simulink model "UAV3D_visualizeBoxObstacle"  (Simulink 8.6)
settings: Solver=ode1  StartTime=0.0  StopTime=inf  FixedStep=1/100  RelTol=1e-6
libraries: uavsimBlockset_UAV3D_visualizeBox x2
settings Model: Creator=j.bolting  LastModifiedBy=j.bolting
settings SolverCC: AutoInsertRateTranBlk=on
settings DataIOCC: SaveFormat=Dataset  SignalLoggingSaveFormat=Dataset
settings OptimizationCC: ExpressionDepthLimit=128
settings DebuggingCC: UnderspecifiedInitializationDetection=Simplified  MergeDetectMultiDrivingBlocksExec=error  SolverPrmCheckMsg=none  FcnCallInpInsideContextMsg=EnableAllAsError  StateNameClashWarn=none
settings HardwareCC: ProdBitPerPointer=64  ProdLargestAtomicFloat=Float  ProdIntDivRoundTo=Zero  ProdEndianess=LittleEndian  ProdWordSize=64  ProdHWDeviceType=Intel->x86-64 (Windows64)
settings GRTTargetCC: GeneratePreprocessorConditionals=Use local settings  CombineOutputUpdateFcns=on  GRTInterface=off
settings ConfigComp: CovModelRefEnable=off

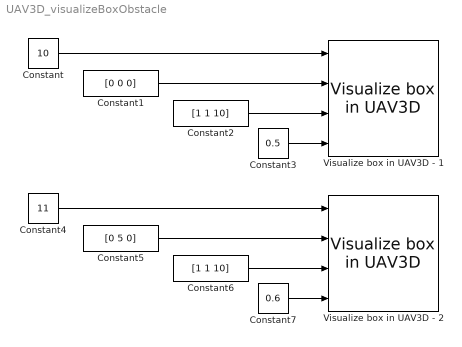
== system UAV3D_visualizeBoxObstacle ==
  Constant : Constant  Value=10
  Constant1 : Constant  Value=[0 0 0]
  Constant2 : Constant  Value=[1 1 10]
  Constant3 : Constant  Value=0.5
  Constant4 : Constant  Value=11
  Constant5 : Constant  Value=[0 5 0]
  Constant6 : Constant  Value=[1 1 10]
  Constant7 : Constant  Value=0.6
  Visualize box in UAV3D - 1 : uavsimBlockset_UAV3D_visualizeBox/Visualize box in UAV3D
  Visualize box in UAV3D - 2 : uavsimBlockset_UAV3D_visualizeBox/Visualize box in UAV3D
  wires:
  Constant/1 -> Visualize box in UAV3D - 1/1
  Constant1/1 -> Visualize box in UAV3D - 1/2
  Constant2/1 -> Visualize box in UAV3D - 1/3
  Constant3/1 -> Visualize box in UAV3D - 1/4
  Constant4/1 -> Visualize box in UAV3D - 2/1
  Constant5/1 -> Visualize box in UAV3D - 2/2
  Constant6/1 -> Visualize box in UAV3D - 2/3
  Constant7/1 -> Visualize box in UAV3D - 2/4
